simulink model "model_moment_bierny"  (Simulink 8.9)
settings: Solver=ode3  StartTime=0.0  StopTime=10  FixedStep=0.006  RelTol=1e-3  EnableMultiTasking=on
undefined symbols (not defined in the file): In, J, Kp, Kt, Kw, lambdan, m, Mn, omegan, psien, R, T, Tp, TR, Un, Uz0, V, Y
settings Model: Creator=Konrad  LastModifiedBy=a
settings OptimizationCC: ExpressionDepthLimit=2147483647
settings DebuggingCC: SolverPrmCheckMsg=warning

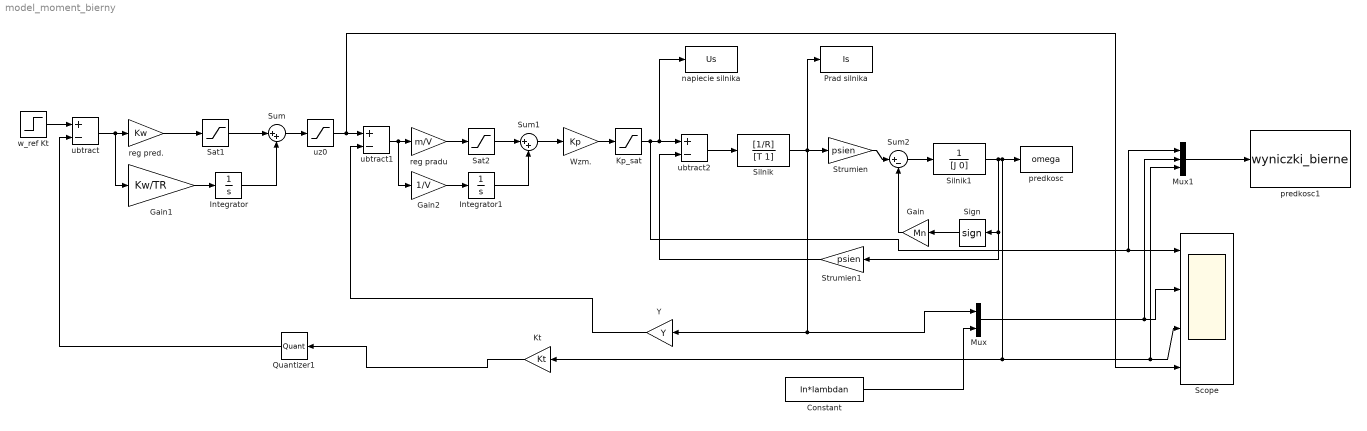
== system model_moment_bierny ==
  Constant : Constant  Value=In*lambdan
  Gain : Gain  Gain=Mn
  Gain1 : Gain  Gain=Kw/TR
  Gain2 : Gain  Gain=1/V
  Integrator : Integrator  LimitOutput=on  UpperSaturationLimit=10  LowerSaturationLimit=-10
  Integrator1 : Integrator  LimitOutput=on  UpperSaturationLimit=10  LowerSaturationLimit=-10
  Kp_sat : Saturate  UpperLimit=1.5*Un  LowerLimit=-1.5*Un
  Kt : Gain  Gain=Kt
  Mux : Mux  Inputs=2
  Mux1 : Mux  Inputs=3
  Prad silnika : ToWorkspace  VariableName=Is  SaveFormat=Structure  SampleTime=-1
  Quantizer1 : Quantizer  QuantizationInterval=123*Tp
  Sat1 : Saturate  UpperLimit=10  LowerLimit=-10
  Sat2 : Saturate  UpperLimit=10  LowerLimit=-10
  Scope : Scope  NumInputPorts=4
  Sign : Signum
  Silnik : TransferFcn  Numerator=[1/R]  Denominator=[T 1]
  Silnik1 : TransferFcn  Denominator=[J 0]
  Strumien : Gain  Gain=psien
  Strumien1 : Gain  Gain=psien
  Sum : Sum  Inputs=|++
  Sum1 : Sum  Inputs=|++
  Sum2 : Sum  Inputs=|+-
  Wzm. : Gain  Gain=Kp
  Y : Gain  Gain=Y
  napiecie silnika : ToWorkspace  VariableName=Us  SaveFormat=Structure  SampleTime=-1
  predkosc : ToWorkspace  VariableName=omega  SaveFormat=Structure  SampleTime=-1
  predkosc1 : ToWorkspace  VariableName=wyniczki_bierne  SaveFormat=Structure With Time  SampleTime=-1
  reg pradu : Gain  Gain=m/V
  reg pred. : Gain  Gain=Kw
  ubtract : Sum  Inputs=+-
  ubtract1 : Sum  Inputs=+-
  ubtract2 : Sum  Inputs=+-
  uz0 : Saturate  UpperLimit=Uz0  LowerLimit=-Uz0
  w_ref Kt : Step  Time=0  After=omegan*Kt  SampleTime=0
  wires:
  w_ref Kt/1 -> ubtract/1
  ubtract/1 -> reg pred./1, Gain1/1
  reg pred./1 -> Sat1/1
  Sat1/1 -> Sum/1
  Gain1/1 -> Integrator/1
  Integrator/1 -> Sum/2
  Sum/1 -> uz0/1
  uz0/1 -> ubtract1/1, Scope/4
  ubtract1/1 -> reg pradu/1, Gain2/1
  reg pradu/1 -> Sat2/1
  Sat2/1 -> Sum1/1
  Gain2/1 -> Integrator1/1
  Integrator1/1 -> Sum1/2
  Sum1/1 -> Wzm./1
  Wzm./1 -> Kp_sat/1
  Kp_sat/1 -> ubtract2/1, napiecie silnika/1, Mux1/1, Scope/1
  ubtract2/1 -> Silnik/1
  Silnik/1 -> Strumien/1, Prad silnika/1, Mux/1, Y/1
  Strumien/1 -> Sum2/1
  Sum2/1 -> Silnik1/1
  Silnik1/1 -> predkosc/1, Scope/3, Mux1/3, Kt/1, Strumien1/1, Sign/1
  Mux/1 -> Mux1/2, Scope/2
  Strumien1/1 -> ubtract2/2
  Constant/1 -> Mux/2
  Gain/1 -> Sum2/2
  Sign/1 -> Gain/1
  Mux1/1 -> predkosc1/1
  Quantizer1/1 -> ubtract/2
  Y/1 -> ubtract1/2
  Kt/1 -> Quantizer1/1
